simulink model "e1"  (R2017a)
settings: Solver=FixedStepAuto  StartTime=0.0  StopTime=10.0  FixedStep=0.1  RelTol=1e-3
settings Model: Creator=Soutrik  LastModifiedBy=Soutrik

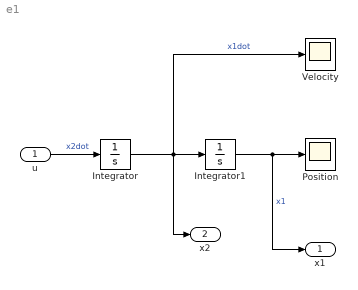
== system e1 ==
  u : Inport
  Integrator : Integrator
  Integrator1 : Integrator
  Position : Scope
  Velocity : Scope
  x1 : Outport
  x2 : Outport  Port=2
  wires:
  u/1 -> Integrator/1  "x2dot"
  Integrator/1 -> Velocity/1, Integrator1/1, x2/1  "x1dot"
  Integrator1/1 -> x1/1, Position/1  "x1"
